simulink model "architecture1"  (R2019b)
settings: Solver=VariableStepAuto  StartTime=0.0  StopTime=10.0  RelTol=1e-3
libraries: xbsIndex_r4 x1962
settings Model: Creator=s4533087  LastModifiedBy=s4533087

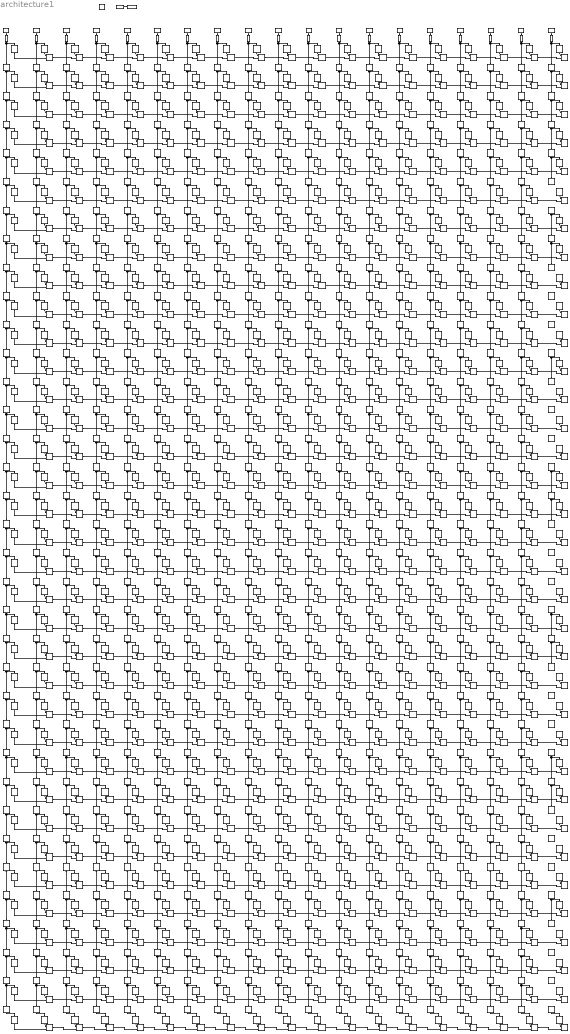
== system architecture1 ==
  " System Generator" : xbsIndex_r4/ System Generator  Tag=genX  xilinxfamily=Kintex7  part=xc7k325t  speed=-3  package=fbg676  synthesis_tool=Vivado  clock_wrapper=Clock Enables  directory=./netlist  proj_type=Vivado  Synth_file=Vivado Synthesis Defaults  Impl_file=Vivado Implementation Defaults  testbench=off  simulink_period=1  sysclk_period=10  dcm_input_clock_period=10  incr_netlist=off  trim_vbits=Everywhere in SubSystem  dbl_ovrd=According to Block Masks  core_generation=According to Block Masks  run_coregen=off  deprecated_control=off  eval_field=0  block_type=sysgen
  AddSub{1..630} (630 alike) : xbsIndex_r4/AddSub  mode=Addition  use_carryin=off  use_carryout=off  en=off  latency=0  precision=Full  arith_type=Unsigned  n_bits=16  bin_pt=14  quantization=Truncate  overflow=Wrap  use_behavioral_HDL=off  hw_selection=Fabric  pipelined=off  dbl_ovrd=off  block_type=addsub
  CMult{,1..664} (665 alike) : xbsIndex_r4/CMult  const=1  gui_display_data_type=Fixed-point  const_n_bits=16  const_bin_pt=14  float_type=Single  exp_bits=8  fraction_bits=24  en=off  latency=0  precision=User Defined  arith_type="Signed  (2's comp)"  n_bits=Wc  bin_pt=Dc  quantization=Truncate  overflow=Flag as error  use_behavioral_HDL=off  mem_type=Distributed RAM  pipeline=off  dbl_ovrd=off  block_type=cmult
  Delay{,1..645} (646 alike) : xbsIndex_r4/Delay  rst=off  infoeditControl=Selection of Reset will increase slice count due to use of real FFs and instead of SRLs  en=off  latency=1  reg_retiming=off  dbl_ovrd=off  block_type=delay
  From Workspace : FromWorkspace  VariableName=sig(:, 1)  SampleTime=0
  From Workspace1 : FromWorkspace  VariableName=sig(:, 2)  SampleTime=0
  From Workspace{2,4,6,8,10,12,14,16} (8 alike) : FromWorkspace  VariableName=sig(:, 3)  SampleTime=0
  From Workspace{3,5,7,9,11,13,15,17..18} (9 alike) : FromWorkspace  VariableName=sig(:, 4)  SampleTime=0
  Gateway In{,1..18} (19 alike) : xbsIndex_r4/Gateway In  gui_display_data_type=Fixed-point  arith_type="Signed  (2's comp)"  n_bits=W  bin_pt=D  preci_type=Single  exp_width=8  frac_width=24  rows=1  columns=1  quantization="Round  (unbiased: +/- Inf)"  overflow=Saturate  period=1  UseAsADC=off  ADCChannel='1'  interface=None  automatic_assignment=on  address_offset=hex2dec('00')  intf_name=''  intf_description=''  default_value=0  timing_constraint=None  locs_specified=off  LOCs={}  io_standard={}  inherit_from_input=off  hdl_port=on  dbl_ovrd=off  block_type=gatewayin
  Gateway Out : xbsIndex_r4/Gateway Out  inherit_from_input=off  hdl_port=on  rows=1  columns=1  UseAsDAC=off  DACChannel='1'  interface=None  automatic_assignment=on  address_offset=hex2dec('00')  intf_name=''  intf_description=''  timing_constraint=None  locs_specified=off  LOCs={}  io_standard={}  block_type=gatewayout
  To Workspace : ToWorkspace  VariableName=simout  SaveFormat=Timeseries  SampleTime=-1
  wires:
  From Workspace/1 -> Gateway In/1
  Gateway Out/1 -> To Workspace/1
  Gateway In/1 -> CMult/1, Delay/1
  Delay/1 -> CMult1/1, Delay1/1
  Delay1/1 -> CMult2/1, Delay2/1
  Delay2/1 -> CMult3/1, Delay3/1
  Delay3/1 -> CMult4/1, Delay4/1
  Delay4/1 -> CMult5/1, Delay5/1
  Delay8/1 -> CMult9/1, Delay9/1
  Delay10/1 -> CMult11/1, Delay11/1
  Delay6/1 -> CMult7/1, Delay7/1
  Delay7/1 -> CMult8/1, Delay8/1
  Delay5/1 -> CMult6/1, Delay6/1
  Delay9/1 -> CMult10/1, Delay10/1
  Delay16/1 -> CMult12/1, Delay12/1
  Delay12/1 -> CMult13/1, Delay13/1
  Delay11/1 -> CMult14/1, Delay14/1
  Delay14/1 -> CMult15/1, Delay15/1
  Delay15/1 -> CMult16/1, Delay16/1
  Delay20/1 -> CMult23/1, Delay23/1
  Delay31/1 -> CMult32/1, Delay32/1
  Delay32/1 -> CMult33/1, Delay33/1
  Delay19/1 -> CMult20/1, Delay20/1
  Delay28/1 -> CMult29/1, Delay29/1
  Delay33/1 -> CMult19/1, Delay19/1
  Delay29/1 -> CMult30/1, Delay30/1
  Delay17/1 -> CMult18/1, Delay18/1
  Delay18/1 -> CMult26/1, Delay26/1
  Delay13/1 -> CMult17/1, Delay17/1
  Delay26/1 -> CMult27/1, Delay27/1
  Delay25/1 -> CMult21/1, Delay21/1
  Delay21/1 -> CMult22/1, Delay22/1
  Delay24/1 -> CMult25/1, Delay25/1
  Delay30/1 -> CMult31/1, Delay31/1
  Delay23/1 -> CMult24/1, Delay24/1
  Delay27/1 -> CMult28/1, Delay28/1
  Delay22/1 -> CMult34/1
  Delay39/1 -> CMult44/1, Delay43/1
  CMult63/1 -> AddSub63/1
  Delay37/1 -> CMult41/1, Delay40/1
  CMult66/1 -> AddSub66/1
  CMult68/1 -> AddSub68/1
  CMult69/1 -> AddSub69/1
  Delay36/1 -> CMult38/1, Delay37/1
  Delay64/1 -> CMult67/1, Delay65/1
  CMult37/1 -> AddSub37/1
  Delay65/1 -> CMult68/1, Delay66/1
  Delay66/1 -> CMult69/1, Delay67/1
  CMult38/1 -> AddSub38/1
  Delay57/1 -> CMult64/1, Delay62/1
  CMult65/1 -> AddSub65/1
  Delay62/1 -> CMult65/1, Delay63/1
  CMult64/1 -> AddSub64/1
  CMult40/1 -> AddSub40/1
  Delay67/1 -> CMult37/1, Delay36/1
  Delay41/1 -> CMult43/1, Delay42/1
  CMult67/1 -> AddSub67/1
  Delay40/1 -> CMult42/1, Delay41/1
  CMult39/1 -> AddSub39/1
  Delay63/1 -> CMult66/1, Delay64/1
  Delay35/1 -> CMult47/1, Delay46/1
  CMult36/1 -> AddSub36/1
  Delay49/1 -> CMult63/1
  Delay34/1 -> CMult36/1, Delay35/1
  Gateway In1/1 -> CMult35/1, Delay34/1
  Delay42/1 -> CMult39/1, Delay38/1
  Delay38/1 -> CMult40/1, Delay39/1
  From Workspace1/1 -> Gateway In1/1
  CMult47/1 -> AddSub47/1
  CMult41/1 -> AddSub41/1
  CMult59/1 -> AddSub59/1
  CMult46/1 -> AddSub46/1
  Delay56/1 -> CMult59/1, Delay58/1
  CMult45/1 -> AddSub45/1
  CMult50/1 -> AddSub50/1
  Delay61/1 -> CMult46/1, Delay45/1
  Delay60/1 -> CMult62/1, Delay61/1
  CMult48/1 -> AddSub48/1
  CMult54/1 -> AddSub54/1
  CMult49/1 -> AddSub49/1
  CMult55/1 -> AddSub55/1
  Delay47/1 -> CMult51/1, Delay50/1
  CMult44/1 -> AddSub44/1
  CMult61/1 -> AddSub61/1
  Delay58/1 -> CMult60/1, Delay59/1
  Delay59/1 -> CMult61/1, Delay60/1
  Delay51/1 -> CMult53/1, Delay52/1
  CMult42/1 -> AddSub42/1
  Delay46/1 -> CMult58/1, Delay57/1
  Delay48/1 -> CMult50/1, Delay49/1
  CMult62/1 -> AddSub62/1
  Delay52/1 -> CMult49/1, Delay48/1
  CMult43/1 -> AddSub43/1
  Delay53/1 -> CMult55/1, Delay54/1
  Delay45/1 -> CMult48/1, Delay47/1
  CMult60/1 -> AddSub60/1
  CMult52/1 -> AddSub52/1
  CMult53/1 -> AddSub53/1
  Delay50/1 -> CMult52/1, Delay51/1
  CMult56/1 -> AddSub56/1
  Delay54/1 -> CMult56/1, Delay55/1
  Delay55/1 -> CMult57/1, Delay56/1
  Delay43/1 -> CMult45/1, Delay44/1
  CMult35/1 -> AddSub35/1
  CMult51/1 -> AddSub51/1
  CMult58/1 -> AddSub58/1
  CMult57/1 -> AddSub57/1
  Delay44/1 -> CMult54/1, Delay53/1
  CMult/1 -> AddSub35/2
  CMult1/1 -> AddSub36/2
  CMult2/1 -> AddSub47/2
  CMult3/1 -> AddSub58/2
  CMult4/1 -> AddSub64/2
  CMult5/1 -> AddSub65/2
  CMult6/1 -> AddSub66/2
  CMult7/1 -> AddSub67/2
  CMult8/1 -> AddSub68/2
  CMult9/1 -> AddSub69/2
  CMult10/1 -> AddSub37/2
  CMult11/1 -> AddSub38/2
  CMult14/1 -> AddSub41/2
  CMult15/1 -> AddSub42/2
  CMult16/1 -> AddSub43/2
  CMult12/1 -> AddSub39/2
  CMult13/1 -> AddSub40/2
  CMult17/1 -> AddSub44/2
  CMult18/1 -> AddSub45/2
  CMult26/1 -> AddSub54/2
  CMult27/1 -> AddSub55/2
  CMult28/1 -> AddSub56/2
  CMult29/1 -> AddSub57/2
  CMult30/1 -> AddSub59/2
  CMult31/1 -> AddSub60/2
  CMult32/1 -> AddSub61/2
  CMult33/1 -> AddSub62/2
  CMult19/1 -> AddSub46/2
  CMult20/1 -> AddSub48/2
  CMult23/1 -> AddSub51/2
  CMult24/1 -> AddSub52/2
  CMult25/1 -> AddSub53/2
  CMult21/1 -> AddSub49/2
  CMult22/1 -> AddSub50/2
  CMult34/1 -> AddSub63/2
  CMult82/1 -> AddSub13/1
  Delay90/1 -> CMult94/1, Delay92/1
  From Workspace2/1 -> Gateway In2/1
  CMult81/1 -> AddSub12/1
  CMult94/1 -> AddSub25/1
  CMult76/1 -> AddSub7/1
  Gateway In2/1 -> CMult70/1, Delay68/1
  Delay72/1 -> CMult75/1, Delay73/1
  Delay76/1 -> CMult74/1, Delay72/1
  Delay97/1 -> CMult101/1, Delay98/1
  Delay68/1 -> CMult71/1, Delay69/1
  CMult71/1 -> AddSub2/1
  Delay69/1 -> CMult82/1, Delay80/1
  Delay83/1 -> CMult98/1
  CMult102/1 -> AddSub33/1
  Delay75/1 -> CMult78/1, Delay76/1
  Delay74/1 -> CMult77/1, Delay75/1
  CMult74/1 -> AddSub5/1
  Delay101/1 -> CMult72/1, Delay70/1
  CMult75/1 -> AddSub6/1
  CMult100/1 -> AddSub31/1
  CMult99/1 -> AddSub30/1
  Delay96/1 -> CMult100/1, Delay97/1
  Delay91/1 -> CMult99/1, Delay96/1
  Delay99/1 -> CMult103/1, Delay100/1
  CMult72/1 -> AddSub3/1
  CMult73/1 -> AddSub4/1
  Delay100/1 -> CMult104/1, Delay101/1
  CMult103/1 -> AddSub34/1
  CMult101/1 -> AddSub32/1
  CMult104/1 -> AddSub70/1
  Delay98/1 -> CMult102/1, Delay99/1
  Delay71/1 -> CMult76/1, Delay74/1
  CMult98/1 -> AddSub29/1
  Delay73/1 -> CMult79/1, Delay77/1
  AddSub35/1 -> AddSub1/2
  CMult97/1 -> AddSub28/1
  Delay86/1 -> CMult84/1, Delay82/1
  Delay80/1 -> CMult93/1, Delay91/1
  Delay92/1 -> CMult95/1, Delay93/1
  CMult77/1 -> AddSub8/1
  Delay81/1 -> CMult86/1, Delay84/1
  CMult83/1 -> AddSub14/1
  CMult84/1 -> AddSub15/1
  CMult79/1 -> AddSub10/1
  CMult89/1 -> AddSub20/1
  CMult90/1 -> AddSub21/1
  Delay95/1 -> CMult81/1, Delay79/1
  CMult80/1 -> AddSub11/1
  Delay78/1 -> CMult89/1, Delay87/1
  CMult92/1 -> AddSub23/1
  CMult70/1 -> AddSub1/1
  CMult85/1 -> AddSub16/1
  CMult93/1 -> AddSub24/1
  Delay77/1 -> CMult80/1, Delay78/1
  Delay85/1 -> CMult88/1, Delay86/1
  Delay94/1 -> CMult97/1, Delay95/1
  Delay84/1 -> CMult87/1, Delay85/1
  Delay82/1 -> CMult85/1, Delay83/1
  Delay88/1 -> CMult91/1, Delay89/1
  CMult91/1 -> AddSub22/1
  Delay89/1 -> CMult92/1, Delay90/1
  Delay79/1 -> CMult83/1, Delay81/1
  Delay87/1 -> CMult90/1, Delay88/1
  Delay70/1 -> CMult73/1, Delay71/1
  CMult88/1 -> AddSub19/1
  CMult78/1 -> AddSub9/1
  CMult95/1 -> AddSub26/1
  CMult96/1 -> AddSub27/1
  CMult86/1 -> AddSub17/1
  Delay93/1 -> CMult96/1, Delay94/1
  CMult87/1 -> AddSub18/1
  AddSub36/1 -> AddSub2/2
  AddSub47/1 -> AddSub13/2
  AddSub58/1 -> AddSub24/2
  AddSub64/1 -> AddSub30/2
  AddSub65/1 -> AddSub31/2
  AddSub66/1 -> AddSub32/2
  AddSub67/1 -> AddSub33/2
  AddSub68/1 -> AddSub34/2
  AddSub69/1 -> AddSub70/2
  AddSub37/1 -> AddSub3/2
  AddSub38/1 -> AddSub4/2
  AddSub41/1 -> AddSub7/2
  AddSub42/1 -> AddSub8/2
  AddSub43/1 -> AddSub9/2
  AddSub39/1 -> AddSub5/2
  AddSub40/1 -> AddSub6/2
  AddSub44/1 -> AddSub10/2
  AddSub45/1 -> AddSub11/2
  AddSub54/1 -> AddSub20/2
  AddSub55/1 -> AddSub21/2
  AddSub56/1 -> AddSub22/2
  AddSub57/1 -> AddSub23/2
  AddSub59/1 -> AddSub25/2
  AddSub60/1 -> AddSub26/2
  AddSub61/1 -> AddSub27/2
  AddSub62/1 -> AddSub28/2
  AddSub46/1 -> AddSub12/2
  AddSub48/1 -> AddSub14/2
  AddSub51/1 -> AddSub17/2
  AddSub52/1 -> AddSub18/2
  AddSub53/1 -> AddSub19/2
  AddSub49/1 -> AddSub15/2
  AddSub50/1 -> AddSub16/2
  AddSub63/1 -> AddSub29/2
  AddSub11/1 -> AddSub73/2
  AddSub21/1 -> AddSub84/2
  AddSub3/1 -> AddSub93/2
  AddSub34/1 -> AddSub98/2
  AddSub10/1 -> AddSub72/2
  AddSub9/1 -> AddSub105/2
  AddSub17/1 -> AddSub79/2
  AddSub14/1 -> AddSub76/2
  AddSub8/1 -> AddSub104/2
  AddSub12/1 -> AddSub74/2
  AddSub15/1 -> AddSub77/2
  Delay126/1 -> CMult134/1, Delay128/1
  CMult122/1 -> AddSub75/1
  CMult134/1 -> AddSub88/1
  AddSub13/1 -> AddSub75/2
  CMult136/1 -> AddSub90/1
  Delay129/1 -> CMult136/1, Delay130/1
  CMult127/1 -> AddSub80/1
  CMult126/1 -> AddSub79/1
  Delay123/1 -> CMult130/1, Delay124/1
  CMult135/1 -> AddSub89/1
  CMult118/1 -> AddSub105/1
  Delay106/1 -> CMult113/1, Delay107/1
  CMult131/1 -> AddSub85/1
  CMult121/1 -> AddSub74/1
  Delay124/1 -> CMult131/1, Delay125/1
  Delay125/1 -> CMult132/1, Delay126/1
  Delay130/1 -> CMult137/1, Delay131/1
  CMult110/1 -> AddSub71/1
  CMult133/1 -> AddSub87/1
  Delay121/1 -> CMult128/1, Delay122/1
  Delay113/1 -> CMult120/1, Delay114/1
  CMult125/1 -> AddSub78/1
  CMult132/1 -> AddSub86/1
  CMult130/1 -> AddSub84/1
  CMult129/1 -> AddSub83/1
  Delay114/1 -> CMult129/1, Delay123/1
  CMult120/1 -> AddSub73/1
  CMult117/1 -> AddSub104/1
  Delay117/1 -> CMult126/1, Delay120/1
  CMult124/1 -> AddSub77/1
  CMult119/1 -> AddSub72/1
  CMult123/1 -> AddSub76/1
  Delay128/1 -> CMult135/1, Delay129/1
  CMult137/1 -> AddSub91/1
  Delay116/1 -> CMult133/1, Delay127/1
  Delay122/1 -> CMult124/1, Delay118/1
  Delay134/1 -> CMult107/1, Delay135/1
  Delay107/1 -> CMult116/1, Delay110/1
  Delay120/1 -> CMult127/1, Delay121/1
  CMult109/1 -> AddSub103/1
  Delay109/1 -> CMult119/1, Delay113/1
  CMult138/1 -> AddSub92/1
  CMult106/1 -> AddSub96/1
  CMult112/1 -> AddSub93/1
  Delay118/1 -> CMult125/1, Delay119/1
  Delay102/1 -> CMult109/1, Delay103/1
  CMult108/1 -> AddSub98/1
  Delay127/1 -> CMult139/1, Delay132/1
  Delay115/1 -> CMult123/1, Delay117/1
  CMult114/1 -> AddSub100/1
  Delay135/1 -> CMult108/1, Delay102/1
  CMult105/1 -> AddSub95/1
  Delay103/1 -> CMult112/1, Delay106/1
  Delay110/1 -> CMult117/1, Delay111/1
  Delay111/1 -> CMult118/1, Delay112/1
  Delay119/1 -> CMult138/1
  Delay104/1 -> CMult111/1, Delay105/1
  Delay132/1 -> CMult105/1, Delay133/1
  CMult111/1 -> AddSub82/1
  Delay112/1 -> CMult114/1, Delay108/1
  Delay108/1 -> CMult115/1, Delay109/1
  CMult113/1 -> AddSub99/1
  AddSub29/1 -> AddSub92/2
  Delay105/1 -> CMult122/1, Delay116/1
  AddSub16/1 -> AddSub78/2
  Gateway In3/1 -> CMult110/1, Delay104/1
  CMult116/1 -> AddSub102/1
  AddSub27/1 -> AddSub90/2
  AddSub30/1 -> AddSub94/2
  CMult128/1 -> AddSub81/1
  AddSub7/1 -> AddSub102/2
  Delay131/1 -> CMult121/1, Delay115/1
  AddSub4/1 -> AddSub99/2
  AddSub20/1 -> AddSub83/2
  AddSub28/1 -> AddSub91/2
  From Workspace3/1 -> Gateway In3/1
  AddSub1/1 -> AddSub71/2
  AddSub22/1 -> AddSub85/2
  AddSub19/1 -> AddSub81/2
  AddSub18/1 -> AddSub80/2
  CMult115/1 -> AddSub101/1
  CMult139/1 -> AddSub94/1
  AddSub31/1 -> AddSub95/2
  AddSub33/1 -> AddSub97/2
  AddSub32/1 -> AddSub96/2
  Delay133/1 -> CMult106/1, Delay134/1
  CMult107/1 -> AddSub97/1
  AddSub25/1 -> AddSub88/2
  AddSub70/1 -> AddSub103/2
  AddSub5/1 -> AddSub100/2
  AddSub24/1 -> AddSub87/2
  AddSub23/1 -> AddSub86/2
  AddSub2/1 -> AddSub82/2
  AddSub26/1 -> AddSub89/2
  AddSub6/1 -> AddSub101/2
  AddSub139/1 -> AddSub174/2
  AddSub135/1 -> AddSub170/2
  AddSub133/1 -> AddSub168/2
  AddSub138/1 -> AddSub173/2
  AddSub131/1 -> AddSub166/2
  AddSub136/1 -> AddSub171/2
  AddSub130/1 -> AddSub164/2
  AddSub127/1 -> AddSub161/2
  AddSub128/1 -> AddSub162/2
  AddSub122/1 -> AddSub156/2
  AddSub124/1 -> AddSub158/2
  AddSub107/1 -> AddSub146/2
  AddSub114/1 -> AddSub147/2
  AddSub142/1 -> AddSub109/2
  AddSub154/1 -> AddSub112/2
  AddSub140/1 -> AddSub175/2
  AddSub73/1 -> AddSub114/2
  AddSub93/1 -> AddSub134/2
  AddSub98/1 -> AddSub139/2
  AddSub126/1 -> AddSub160/2
  AddSub72/1 -> AddSub107/2
  AddSub105/1 -> AddSub165/2
  AddSub79/1 -> AddSub120/2
  AddSub76/1 -> AddSub117/2
  AddSub77/1 -> AddSub118/2
  CMult192/1 -> AddSub116/1
  CMult204/1 -> AddSub129/1
  AddSub75/1 -> AddSub116/2
  CMult206/1 -> AddSub131/1
  Delay197/1 -> CMult206/1, Delay198/1
  CMult197/1 -> AddSub121/1
  CMult196/1 -> AddSub120/1
  Delay191/1 -> CMult200/1, Delay192/1
  CMult205/1 -> AddSub130/1
  CMult188/1 -> AddSub165/1
  CMult201/1 -> AddSub126/1
  CMult191/1 -> AddSub115/1
  Delay192/1 -> CMult201/1, Delay193/1
  Delay193/1 -> CMult202/1, Delay194/1
  AddSub144/1 -> AddSub111/2
  Delay198/1 -> CMult207/1, Delay199/1
  Delay189/1 -> CMult198/1, Delay190/1
  Delay181/1 -> CMult190/1, Delay182/1
  CMult195/1 -> AddSub119/1
  AddSub106/1 -> AddSub145/2
  CMult202/1 -> AddSub127/1
  Delay182/1 -> CMult199/1, Delay191/1
  CMult190/1 -> AddSub114/1
  CMult194/1 -> AddSub118/1
  CMult193/1 -> AddSub117/1
  Delay196/1 -> CMult205/1, Delay197/1
  CMult207/1 -> AddSub132/1
  Delay184/1 -> CMult203/1, Delay195/1
  Delay190/1 -> CMult194/1, Delay186/1
  Delay202/1 -> CMult142/1, Delay203/1
  Delay188/1 -> CMult197/1, Delay189/1
  CMult144/1 -> AddSub144/1
  Delay177/1 -> CMult189/1, Delay181/1
  CMult141/1 -> AddSub137/1
  CMult143/1 -> AddSub139/1
  AddSub119/1 -> AddSub152/2
  CMult183/1 -> AddSub140/1
  Delay203/1 -> CMult143/1, Delay136/1
  Delay200/1 -> CMult140/1, Delay201/1
  AddSub121/1 -> AddSub155/2
  CMult184/1 -> AddSub141/1
  CMult140/1 -> AddSub136/1
  Delay137/1 -> CMult182/1, Delay174/1
  AddSub143/1 -> AddSub110/2
  Delay178/1 -> CMult187/1, Delay179/1
  Delay187/1 -> CMult208/1
  Delay172/1 -> CMult181/1, Delay173/1
  CMult181/1 -> AddSub123/1
  Delay173/1 -> CMult192/1, Delay184/1
  Delay176/1 -> CMult185/1, Delay177/1
  AddSub116/1 -> AddSub149/2
  AddSub92/1 -> AddSub133/2
  Delay201/1 -> CMult141/1, Delay202/1
  AddSub85/1 -> AddSub126/2
  AddSub101/1 -> AddSub142/2
  AddSub78/1 -> AddSub119/2
  Delay159/1 -> CMult170/1, Delay160/1
  Delay166/1 -> CMult177/1, Delay167/1
  AddSub137/1 -> AddSub172/2
  AddSub71/1 -> AddSub106/2
  Delay161/1 -> CMult172/1, Delay162/1
  AddSub104/1 -> AddSub154/2
  Delay160/1 -> CMult171/1, Delay161/1
  CMult161/1 -> AddSub148/1
  Delay194/1 -> CMult204/1, Delay196/1
  CMult171/1 -> AddSub160/1
  Delay142/1 -> CMult153/1, Delay143/1
  CMult208/1 -> AddSub133/1
  AddSub117/1 -> AddSub150/2
  CMult158/1 -> AddSub113/1
  CMult175/1 -> AddSub164/1
  Delay136/1 -> CMult144/1, Delay137/1
  CMult173/1 -> AddSub162/1
  CMult150/1 -> AddSub145/1
  CMult160/1 -> AddSub147/1
  Delay185/1 -> CMult196/1, Delay188/1
  Delay179/1 -> CMult188/1, Delay180/1
  AddSub132/1 -> AddSub167/2
  CMult169/1 -> AddSub158/1
  CMult180/1 -> AddSub106/1
  AddSub129/1 -> AddSub163/2
  CMult170/1 -> AddSub159/1
  CMult172/1 -> AddSub161/1
  CMult165/1 -> AddSub152/1
  Delay149/1 -> CMult160/1, Delay150/1
  AddSub90/1 -> AddSub131/2
  Delay157/1 -> CMult168/1, Delay158/1
  Delay175/1 -> CMult186/1, Delay178/1
  Gateway In4/1 -> CMult180/1, Delay172/1
  CMult186/1 -> AddSub143/1
  AddSub94/1 -> AddSub135/2
  CMult198/1 -> AddSub122/1
  AddSub102/1 -> AddSub143/2
  Delay199/1 -> CMult191/1, Delay183/1
  AddSub99/1 -> AddSub140/2
  AddSub83/1 -> AddSub124/2
  AddSub91/1 -> AddSub132/2
  From Workspace4/1 -> Gateway In4/1
  AddSub81/1 -> AddSub122/2
  AddSub80/1 -> AddSub121/2
  CMult147/1 -> AddSub173/1
  CMult200/1 -> AddSub125/1
  CMult155/1 -> AddSub109/1
  Delay171/1 -> CMult148/1, Delay138/1
  CMult154/1 -> AddSub108/1
  Delay151/1 -> CMult163/1, Delay153/1
  AddSub74/1 -> AddSub115/2
  CMult182/1 -> AddSub134/1
  Delay186/1 -> CMult195/1, Delay187/1
  AddSub95/1 -> AddSub136/2
  AddSub89/1 -> AddSub130/2
  Delay150/1 -> CMult169/1, Delay159/1
  AddSub86/1 -> AddSub127/2
  Delay163/1 -> CMult179/1, Delay168/1
  AddSub96/1 -> AddSub137/2
  CMult148/1 -> AddSub174/1
  CMult142/1 -> AddSub138/1
  Delay138/1 -> CMult149/1, Delay139/1
  AddSub115/1 -> AddSub148/2
  CMult178/1 -> AddSub168/1
  AddSub97/1 -> AddSub138/2
  CMult152/1 -> AddSub169/1
  CMult146/1 -> AddSub172/1
  CMult149/1 -> AddSub111/1
  Delay156/1 -> CMult167/1, Delay157/1
  AddSub123/1 -> AddSub157/2
  AddSub88/1 -> AddSub129/2
  Delay143/1 -> CMult156/1, Delay146/1
  CMult189/1 -> AddSub107/1
  AddSub103/1 -> AddSub144/2
  Delay170/1 -> CMult147/1, Delay171/1
  CMult145/1 -> AddSub171/1
  AddSub134/1 -> AddSub169/2
  AddSub165/1 -> AddSub113/2
  Delay140/1 -> CMult151/1, Delay141/1
  Delay180/1 -> CMult184/1, Delay176/1
  Delay146/1 -> CMult157/1, Delay147/1
  Gateway In5/1 -> CMult150/1, Delay140/1
  CMult179/1 -> AddSub170/1
  AddSub141/1 -> AddSub108/2
  CMult153/1 -> AddSub175/1
  AddSub84/1 -> AddSub125/2
  CMult187/1 -> AddSub154/1
  Delay144/1 -> CMult155/1, Delay145/1
  Delay141/1 -> CMult162/1, Delay152/1
  Delay168/1 -> CMult145/1, Delay169/1
  CMult168/1 -> AddSub156/1
  CMult209/1 -> AddSub135/1
  CMult156/1 -> AddSub110/1
  CMult185/1 -> AddSub142/1
  AddSub120/1 -> AddSub153/2
  Delay155/1 -> CMult178/1
  AddSub82/1 -> AddSub123/2
  CMult174/1 -> AddSub163/1
  Delay183/1 -> CMult193/1, Delay185/1
  CMult162/1 -> AddSub149/1
  Delay169/1 -> CMult146/1, Delay170/1
  Delay162/1 -> CMult174/1, Delay164/1
  CMult151/1 -> AddSub157/1
  CMult199/1 -> AddSub124/1
  CMult176/1 -> AddSub166/1
  Delay167/1 -> CMult161/1, Delay151/1
  CMult167/1 -> AddSub155/1
  Delay165/1 -> CMult176/1, Delay166/1
  CMult166/1 -> AddSub153/1
  Delay158/1 -> CMult164/1, Delay154/1
  Delay152/1 -> CMult173/1, Delay163/1
  AddSub87/1 -> AddSub128/2
  Delay148/1 -> CMult154/1, Delay144/1
  Delay195/1 -> CMult209/1, Delay200/1
  CMult177/1 -> AddSub167/1
  AddSub100/1 -> AddSub141/2
  Delay154/1 -> CMult165/1, Delay155/1
  Delay174/1 -> CMult183/1, Delay175/1
  Delay164/1 -> CMult175/1, Delay165/1
  CMult203/1 -> AddSub128/1
  AddSub118/1 -> AddSub151/2
  Delay139/1 -> CMult152/1, Delay142/1
  CMult159/1 -> AddSub146/1
  Delay145/1 -> CMult159/1, Delay149/1
  CMult164/1 -> AddSub151/1
  Delay153/1 -> CMult166/1, Delay156/1
  CMult157/1 -> AddSub112/1
  CMult163/1 -> AddSub150/1
  From Workspace5/1 -> Gateway In5/1
  AddSub125/1 -> AddSub159/2
  Delay147/1 -> CMult158/1, Delay148/1
  AddSub298/1 -> AddSub204/2
  AddSub303/1 -> AddSub209/2
  AddSub299/1 -> AddSub205/2
  AddSub291/1 -> AddSub197/2
  AddSub293/1 -> AddSub200/2
  AddSub295/1 -> AddSub201/2
  AddSub296/1 -> AddSub202/2
  AddSub287/1 -> AddSub193/2
  AddSub290/1 -> AddSub196/2
  AddSub314/1 -> AddSub220/2
  AddSub307/1 -> AddSub213/2
  AddSub310/1 -> AddSub216/2
  AddSub309/1 -> AddSub215/2
  AddSub178/1 -> AddSub223/2
  AddSub315/1 -> AddSub222/2
  AddSub181/1 -> AddSub226/2
  AddSub182/1 -> AddSub237/2
  AddSub308/1 -> AddSub214/2
  Delay287/1 -> CMult303/1, Delay289/1
  AddSub200/1 -> AddSub236/2
  CMult266/1 -> AddSub189/1
  AddSub223/1 -> AddSub186/2
  CMult278/1 -> AddSub239/1
  CMult297/1 -> AddSub237/1
  AddSub279/1 -> AddSub314/2
  AddSub273/1 -> AddSub308/2
  AddSub278/1 -> AddSub313/2
  AddSub271/1 -> AddSub306/2
  AddSub276/1 -> AddSub311/2
  AddSub267/1 -> AddSub301/2
  AddSub268/1 -> AddSub302/2
  AddSub264/1 -> AddSub298/2
  AddSub261/1 -> AddSub295/2
  Delay259/1 -> CMult288/1
  AddSub254/1 -> AddSub293/2
  AddSub265/1 -> AddSub299/2
  AddSub294/1 -> AddSub182/2
  CMult311/1 -> AddSub206/1
  CMult301/1 -> AddSub194/1
  CMult315/1 -> AddSub211/1
  CMult298/1 -> AddSub249/1
  Delay295/1 -> CMult310/1, Delay296/1
  CMult306/1 -> AddSub200/1
  CMult307/1 -> AddSub201/1
  AddSub289/1 -> AddSub195/2
  AddSub206/1 -> AddSub244/2
  AddSub222/1 -> AddSub260/2
  AddSub193/1 -> AddSub229/2
  AddSub204/1 -> AddSub241/2
  AddSub202/1 -> AddSub239/2
  AddSub211/1 -> AddSub248/2
  AddSub207/1 -> AddSub245/2
  AddSub288/1 -> AddSub194/2
  AddSub212/1 -> AddSub250/2
  AddSub214/1 -> AddSub252/2
  Delay298/1 -> CMult314/1, Delay300/1
  Delay264/1 -> CMult281/1, Delay265/1
  Delay263/1 -> CMult280/1, Delay264/1
  Delay280/1 -> CMult295/1, Delay281/1
  Delay277/1 -> CMult302/1, Delay288/1
  Delay282/1 -> CMult297/1, Delay283/1
  CMult250/1 -> AddSub217/1
  Delay291/1 -> CMult318/1
  AddSub198/1 -> AddSub235/2
  CMult293/1 -> AddSub222/1
  Delay307/1 -> CMult253/1, Delay240/1
  AddSub201/1 -> AddSub238/2
  Delay281/1 -> CMult299/1, Delay285/1
  Delay292/1 -> CMult307/1, Delay293/1
  CMult282/1 -> AddSub245/1
  CMult280/1 -> AddSub242/1
  AddSub213/1 -> AddSub251/2
  AddSub185/1 -> AddSub228/2
  Delay246/1 -> CMult263/1, Delay247/1
  AddSub169/1 -> AddSub274/2
  CMult313/1 -> AddSub208/1
  Delay270/1 -> CMult287/1, Delay271/1
  Delay268/1 -> CMult285/1, Delay269/1
  AddSub153/1 -> AddSub254/2
  AddSub150/1 -> AddSub221/2
  AddSub177/1 -> AddSub286/2
  CMult264/1 -> AddSub186/1
  Delay244/1 -> CMult261/1, Delay245/1
  CMult299/1 -> AddSub185/1
  AddSub215/1 -> AddSub253/2
  Delay274/1 -> CMult257/1, Delay275/1
  Delay247/1 -> CMult266/1, Delay250/1
  AddSub188/1 -> AddSub287/2
  AddSub292/1 -> AddSub198/2
  CMult259/1 -> AddSub190/1
  CMult262/1 -> AddSub253/1
  AddSub203/1 -> AddSub240/2
  CMult288/1 -> AddSub252/1
  AddSub194/1 -> AddSub230/2
  AddSub151/1 -> AddSub232/2
  Delay301/1 -> CMult316/1, Delay302/1
  Delay267/1 -> CMult289/1, Delay272/1
  CMult265/1 -> AddSub187/1
  From Workspace8/1 -> Gateway In8/1
  CMult257/1 -> AddSub258/1
  Delay248/1 -> CMult265/1, Delay249/1
  CMult332/1 -> AddSub210/1
  CMult344/1 -> AddSub269/1
  AddSub237/1 -> AddSub191/2
  CMult256/1 -> AddSub257/1
  AddSub184/1 -> AddSub227/2
  AddSub149/1 -> AddSub210/2
  CMult305/1 -> AddSub198/1
  Delay294/1 -> CMult304/1, Delay290/1
  AddSub275/1 -> AddSub310/2
  Delay288/1 -> CMult313/1, Delay299/1
  AddSub282/1 -> AddSub179/2
  CMult303/1 -> AddSub196/1
  AddSub224/1 -> AddSub187/2
  Delay333/1 -> CMult346/1, Delay334/1
  AddSub216/1 -> AddSub255/2
  CMult337/1 -> AddSub261/1
  CMult336/1 -> AddSub254/1
  Delay241/1 -> CMult292/1, Delay278/1
  Delay327/1 -> CMult340/1, Delay328/1
  CMult345/1 -> AddSub270/1
  CMult328/1 -> AddSub305/1
  Delay283/1 -> CMult298/1, Delay284/1
  Delay265/1 -> CMult282/1, Delay266/1
  CMult341/1 -> AddSub266/1
  Delay329/1 -> CMult342/1, Delay330/1
  CMult272/1 -> AddSub231/1
  AddSub284/1 -> AddSub181/2
  Delay297/1 -> CMult312/1, Delay298/1
  Delay334/1 -> CMult347/1, Delay335/1
  CMult268/1 -> AddSub192/1
  CMult260/1 -> AddSub227/1
  AddSub208/1 -> AddSub246/2
  Delay317/1 -> CMult330/1, Delay318/1
  CMult335/1 -> AddSub243/1
  AddSub176/1 -> AddSub285/2
  Delay296/1 -> CMult311/1, Delay297/1
  Delay318/1 -> CMult339/1, Delay327/1
  CMult330/1 -> AddSub188/1
  CMult334/1 -> AddSub232/1
  CMult333/1 -> AddSub221/1
  Delay332/1 -> CMult345/1, Delay333/1
  AddSub301/1 -> AddSub207/2
  CMult263/1 -> AddSub260/1
  CMult252/1 -> AddSub219/1
  CMult347/1 -> AddSub272/1
  Delay320/1 -> CMult343/1, Delay331/1
  Delay284/1 -> CMult294/1, Delay280/1
  AddSub285/1 -> AddSub184/2
  Delay253/1 -> CMult270/1, Delay254/1
  Delay326/1 -> CMult334/1, Delay322/1
  Delay338/1 -> CMult212/1, Delay339/1
  CMult214/1 -> AddSub284/1
  Delay313/1 -> CMult329/1, Delay317/1
  CMult211/1 -> AddSub277/1
  Delay303/1 -> CMult301/1, Delay287/1
  CMult213/1 -> AddSub279/1
  AddSub243/1 -> AddSub292/2
  CMult323/1 -> AddSub280/1
  Delay336/1 -> CMult210/1, Delay337/1
  Delay260/1 -> CMult277/1, Delay261/1
  CMult324/1 -> AddSub281/1
  AddSub297/1 -> AddSub203/2
  CMult210/1 -> AddSub276/1
  Delay205/1 -> CMult322/1, Delay310/1
  AddSub283/1 -> AddSub180/2
  Delay314/1 -> CMult327/1, Delay315/1
  Delay323/1 -> CMult348/1
  Delay308/1 -> CMult321/1, Delay309/1
  CMult321/1 -> AddSub263/1
  Delay309/1 -> CMult332/1, Delay320/1
  Delay251/1 -> CMult268/1, Delay252/1
  AddSub183/1 -> AddSub249/2
  AddSub195/1 -> AddSub231/2
  Delay312/1 -> CMult325/1, Delay313/1
  AddSub210/1 -> AddSub289/2
  AddSub313/1 -> AddSub219/2
  Delay337/1 -> CMult211/1, Delay338/1
  CMult312/1 -> AddSub207/1
  Delay278/1 -> CMult293/1, Delay279/1
  AddSub160/1 -> AddSub266/2
  AddSub220/1 -> AddSub259/2
  AddSub109/1 -> AddSub282/2
  AddSub249/1 -> AddSub192/2
  AddSub152/1 -> AddSub243/2
  Delay227/1 -> CMult240/1, Delay228/1
  Delay272/1 -> CMult255/1, Delay273/1
  AddSub311/1 -> AddSub217/2
  Delay234/1 -> CMult247/1, Delay235/1
  AddSub277/1 -> AddSub312/2
  AddSub145/1 -> AddSub176/2
  CMult251/1 -> AddSub218/1
  Delay229/1 -> CMult242/1, Delay230/1
  Delay302/1 -> CMult317/1, Delay303/1
  AddSub219/1 -> AddSub258/2
  AddSub304/1 -> AddSub211/2
  Delay228/1 -> CMult241/1, Delay229/1
  Delay290/1 -> CMult305/1, Delay291/1
  Delay330/1 -> CMult344/1, Delay332/1
  CMult241/1 -> AddSub300/1
  CMult255/1 -> AddSub256/1
  CMult348/1 -> AddSub273/1
  Delay210/1 -> CMult223/1, Delay211/1
  CMult253/1 -> AddSub220/1
  CMult228/1 -> AddSub183/1
  CMult245/1 -> AddSub304/1
  Delay204/1 -> CMult214/1, Delay205/1
  CMult243/1 -> AddSub302/1
  CMult220/1 -> AddSub285/1
  AddSub180/1 -> AddSub225/2
  CMult230/1 -> AddSub287/1
  Delay321/1 -> CMult336/1, Delay324/1
  Delay315/1 -> CMult328/1, Delay316/1
  AddSub272/1 -> AddSub307/2
  CMult302/1 -> AddSub195/1
  CMult320/1 -> AddSub176/1
  AddSub269/1 -> AddSub303/2
  Delay306/1 -> CMult252/1, Delay307/1
  CMult239/1 -> AddSub298/1
  CMult240/1 -> AddSub299/1
  CMult294/1 -> AddSub223/1
  CMult235/1 -> AddSub292/1
  CMult285/1 -> AddSub248/1
  Delay217/1 -> CMult230/1, Delay218/1
  Delay250/1 -> CMult267/1, Delay251/1
  AddSub306/1 -> AddSub212/2
  AddSub166/1 -> AddSub271/2
  Delay311/1 -> CMult326/1, Delay314/1
  Delay225/1 -> CMult238/1, Delay226/1
  Gateway In6/1 -> CMult320/1, Delay308/1
  Delay285/1 -> CMult300/1, Delay286/1
  CMult326/1 -> AddSub283/1
  AddSub226/1 -> AddSub190/2
  CMult254/1 -> AddSub226/1
  Delay249/1 -> CMult269/1, Delay253/1
  CMult274/1 -> AddSub234/1
  AddSub209/1 -> AddSub247/2
  AddSub170/1 -> AddSub275/2
  CMult338/1 -> AddSub262/1
  AddSub110/1 -> AddSub283/2
  Delay335/1 -> CMult331/1, Delay319/1
  AddSub175/1 -> AddSub280/2
  AddSub158/1 -> AddSub264/2
  AddSub167/1 -> AddSub272/2
  From Workspace6/1 -> Gateway In6/1
  AddSub179/1 -> AddSub224/2
  AddSub156/1 -> AddSub262/2
  Gateway In9/1 -> CMult260/1, Delay244/1
  CMult217/1 -> AddSub313/1
  CMult340/1 -> AddSub265/1
  CMult225/1 -> AddSub179/1
  Delay239/1 -> CMult218/1, Delay206/1
  CMult224/1 -> AddSub178/1
  Delay219/1 -> CMult233/1, Delay221/1
  AddSub148/1 -> AddSub199/2
  CMult322/1 -> AddSub274/1
  Delay322/1 -> CMult335/1, Delay323/1
  AddSub171/1 -> AddSub276/2
  AddSub164/1 -> AddSub270/2
  Delay286/1 -> CMult309/1, Delay295/1
  Delay218/1 -> CMult239/1, Delay227/1
  AddSub161/1 -> AddSub267/2
  Delay231/1 -> CMult249/1, Delay236/1
  CMult281/1 -> AddSub244/1
  AddSub172/1 -> AddSub277/2
  Delay206/1 -> CMult219/1, Delay207/1
  AddSub199/1 -> AddSub288/2
  CMult248/1 -> AddSub308/1
  AddSub173/1 -> AddSub278/2
  CMult222/1 -> AddSub309/1
  AddSub302/1 -> AddSub208/2
  CMult270/1 -> AddSub229/1
  CMult216/1 -> AddSub312/1
  CMult219/1 -> AddSub181/1
  Delay224/1 -> CMult237/1, Delay225/1
  CMult304/1 -> AddSub197/1
  AddSub263/1 -> AddSub297/2
  AddSub163/1 -> AddSub269/2
  CMult329/1 -> AddSub177/1
  Delay211/1 -> CMult226/1, Delay214/1
  CMult291/1 -> AddSub203/1
  CMult295/1 -> AddSub224/1
  AddSub111/1 -> AddSub284/2
  Delay238/1 -> CMult217/1, Delay239/1
  AddSub312/1 -> AddSub218/2
  CMult249/1 -> AddSub310/1
  AddSub281/1 -> AddSub178/2
  CMult215/1 -> AddSub311/1
  AddSub274/1 -> AddSub309/2
  Delay207/1 -> CMult222/1, Delay210/1
  AddSub305/1 -> AddSub183/2
  Delay208/1 -> CMult221/1, Delay209/1
  Delay316/1 -> CMult324/1, Delay312/1
  Delay214/1 -> CMult227/1, Delay215/1
  Gateway In7/1 -> CMult220/1, Delay208/1
  Delay305/1 -> CMult251/1, Delay306/1
  Delay209/1 -> CMult232/1, Delay220/1
  AddSub232/1 -> AddSub291/2
  CMult325/1 -> AddSub282/1
  CMult226/1 -> AddSub180/1
  CMult223/1 -> AddSub315/1
  AddSub159/1 -> AddSub265/2
  CMult327/1 -> AddSub294/1
  Delay212/1 -> CMult225/1, Delay213/1
  Delay236/1 -> CMult215/1, Delay237/1
  AddSub218/1 -> AddSub257/2
  Delay235/1 -> CMult231/1, Delay219/1
  CMult275/1 -> AddSub235/1
  CMult284/1 -> AddSub247/1
  CMult349/1 -> AddSub275/1
  CMult238/1 -> AddSub296/1
  AddSub196/1 -> AddSub233/2
  CMult289/1 -> AddSub255/1
  AddSub217/1 -> AddSub256/2
  Delay240/1 -> CMult254/1, Delay241/1
  Delay273/1 -> CMult256/1, Delay274/1
  AddSub112/1 -> AddSub294/2
  Delay275/1 -> CMult258/1, Delay242/1
  Delay266/1 -> CMult284/1, Delay268/1
  AddSub266/1 -> AddSub300/2
  AddSub174/1 -> AddSub279/2
  CMult316/1 -> AddSub212/1
  CMult314/1 -> AddSub209/1
  CMult310/1 -> AddSub205/1
  Delay324/1 -> CMult337/1, Delay325/1
  CMult277/1 -> AddSub238/1
  Delay271/1 -> CMult271/1, Delay255/1
  Delay328/1 -> CMult341/1, Delay329/1
  CMult286/1 -> AddSub250/1
  CMult309/1 -> AddSub204/1
  CMult242/1 -> AddSub301/1
  Delay276/1 -> CMult291/1, Delay277/1
  CMult271/1 -> AddSub230/1
  CMult318/1 -> AddSub214/1
  Delay223/1 -> CMult248/1
  Delay215/1 -> CMult228/1, Delay216/1
  CMult244/1 -> AddSub303/1
  Delay319/1 -> CMult333/1, Delay321/1
  AddSub225/1 -> AddSub189/2
  CMult232/1 -> AddSub289/1
  Delay237/1 -> CMult216/1, Delay238/1
  Delay262/1 -> CMult274/1, Delay258/1
  CMult221/1 -> AddSub297/1
  CMult339/1 -> AddSub264/1
  CMult212/1 -> AddSub278/1
  CMult218/1 -> AddSub314/1
  CMult283/1 -> AddSub246/1
  Delay230/1 -> CMult244/1, Delay232/1
  CMult276/1 -> AddSub236/1
  AddSub168/1 -> AddSub273/2
  Delay255/1 -> CMult273/1, Delay257/1
  CMult237/1 -> AddSub295/1
  CMult300/1 -> AddSub193/1
  CMult269/1 -> AddSub228/1
  Delay269/1 -> CMult286/1, Delay270/1
  AddSub197/1 -> AddSub234/2
  CMult317/1 -> AddSub213/1
  AddSub221/1 -> AddSub290/2
  Delay220/1 -> CMult243/1, Delay231/1
  AddSub162/1 -> AddSub268/2
  AddSub108/1 -> AddSub281/2
  AddSub300/1 -> AddSub206/2
  CMult258/1 -> AddSub259/1
  CMult247/1 -> AddSub307/1
  CMult229/1 -> AddSub286/1
  Delay213/1 -> CMult229/1, Delay217/1
  CMult234/1 -> AddSub291/1
  Delay221/1 -> CMult236/1, Delay224/1
  CMult227/1 -> AddSub182/1
  Delay304/1 -> CMult250/1, Delay305/1
  AddSub146/1 -> AddSub177/2
  Delay331/1 -> CMult349/1, Delay336/1
  Delay216/1 -> CMult224/1, Delay212/1
  Delay258/1 -> CMult275/1, Delay259/1
  CMult331/1 -> AddSub199/1
  CMult233/1 -> AddSub290/1
  CMult279/1 -> AddSub241/1
  CMult273/1 -> AddSub233/1
  CMult267/1 -> AddSub191/1
  CMult290/1 -> AddSub184/1
  AddSub270/1 -> AddSub304/2
  Delay222/1 -> CMult235/1, Delay223/1
  Delay293/1 -> CMult308/1, Delay294/1
  Delay310/1 -> CMult323/1, Delay311/1
  CMult292/1 -> AddSub215/1
  Delay257/1 -> CMult276/1, Delay260/1
  Delay226/1 -> CMult234/1, Delay222/1
  AddSub157/1 -> AddSub263/2
  Delay300/1 -> CMult315/1, Delay301/1
  Delay252/1 -> CMult264/1, Delay248/1
  CMult246/1 -> AddSub306/1
  AddSub147/1 -> AddSub188/2
  Delay242/1 -> CMult259/1, Delay243/1
  Delay339/1 -> CMult213/1, Delay204/1
  CMult287/1 -> AddSub251/1
  Delay254/1 -> CMult279/1, Delay263/1
  Delay299/1 -> CMult319/1, Delay304/1
  CMult231/1 -> AddSub288/1
  CMult296/1 -> AddSub225/1
  AddSub280/1 -> AddSub315/2
  CMult236/1 -> AddSub293/1
  CMult319/1 -> AddSub216/1
  Gateway In8/1 -> CMult290/1, Delay276/1
  Delay279/1 -> CMult296/1, Delay282/1
  AddSub262/1 -> AddSub296/2
  Delay232/1 -> CMult245/1, Delay233/1
  CMult343/1 -> AddSub268/1
  Delay261/1 -> CMult278/1, Delay262/1
  Delay233/1 -> CMult246/1, Delay234/1
  CMult342/1 -> AddSub267/1
  CMult261/1 -> AddSub240/1
  AddSub286/1 -> AddSub185/2
  Delay245/1 -> CMult272/1, Delay256/1
  Delay243/1 -> CMult262/1, Delay246/1
  Delay289/1 -> CMult306/1, Delay292/1
  AddSub113/1 -> AddSub305/2
  AddSub155/1 -> AddSub261/2
  Delay256/1 -> CMult283/1, Delay267/1
  Delay325/1 -> CMult338/1, Delay326/1
  CMult308/1 -> AddSub202/1
  From Workspace7/1 -> Gateway In7/1
  CMult346/1 -> AddSub271/1
  From Workspace9/1 -> Gateway In9/1
  AddSub205/1 -> AddSub242/2
  AddSub329/1 -> AddSub520/2
  AddSub331/1 -> AddSub532/2
  AddSub378/1 -> AddSub496/2
  AddSub330/1 -> AddSub521/2
  AddSub371/1 -> AddSub440/2
  AddSub375/1 -> AddSub476/2
  AddSub370/1 -> AddSub426/2
  AddSub384/1 -> AddSub501/2
  AddSub395/1 -> AddSub511/2
  AddSub393/1 -> AddSub510/2
  AddSub397/1 -> AddSub513/2
  AddSub388/1 -> AddSub506/2
  AddSub386/1 -> AddSub503/2
  AddSub391/1 -> AddSub508/2
  AddSub379/1 -> AddSub497/2
  AddSub396/1 -> AddSub512/2
  AddSub392/1 -> AddSub509/2
  AddSub368/1 -> AddSub402/2
  AddSub332/1 -> AddSub545/2
  AddSub434/1 -> AddSub475/2
  From Workspace17/1 -> Gateway In17/1
  From Workspace15/1 -> Gateway In15/1
  Delay496/1 -> CMult533/1, Delay507/1
  CMult558/1 -> AddSub431/1
  AddSub387/1 -> AddSub504/2
  Delay483/1 -> CMult512/1, Delay486/1
  AddSub523/1 -> AddSub411/2
  Delay529/1 -> CMult556/1, Delay532/1
  Delay472/1 -> CMult495/1, Delay473/1
  Delay473/1 -> CMult496/1, Delay474/1
  CMult593/1 -> AddSub503/1
  CMult486/1 -> AddSub531/1
  Delay519/1 -> CMult546/1, Delay522/1
  Gateway In16/1 -> CMult540/1, Delay516/1
  CMult546/1 -> AddSub456/1
  Delay539/1 -> CMult569/1, Delay544/1
  Delay494/1 -> CMult529/1, Delay503/1
  CMult537/1 -> AddSub485/1
  Delay482/1 -> CMult509/1, Delay483/1
  Delay579/1 -> CMult463/1, Delay444/1
  Delay462/1 -> CMult485/1, Delay463/1
  CMult529/1 -> AddSub474/1
  CMult517/1 -> AddSub418/1
  CMult581/1 -> AddSub426/1
  AddSub506/1 -> AddSub544/2
  Delay498/1 -> CMult525/1, Delay499/1
  Delay453/1 -> CMult479/1, Delay457/1
  CMult477/1 -> AddSub408/1
  CMult508/1 -> AddSub493/1
  AddSub540/1 -> AddSub435/2
  Delay460/1 -> CMult493/1, Delay471/1
  CMult487/1 -> AddSub533/1
  CMult550/1 -> AddSub420/1
  AddSub452/1 -> AddSub528/2
  CMult567/1 -> AddSub443/1
  CMult519/1 -> AddSub459/1
  CMult481/1 -> AddSub525/1
  Delay495/1 -> CMult523/1, Delay497/1
  CMult589/1 -> AddSub499/1
  AddSub517/1 -> AddSub556/2
  CMult471/1 -> AddSub535/1
  Delay477/1 -> CMult466/1, Delay478/1
  AddSub456/1 -> AddSub415/2
  Delay463/1 -> CMult498/1
  CMult494/1 -> AddSub543/1
  Delay455/1 -> CMult478/1, Delay456/1
  CMult536/1 -> AddSub484/1
  CMult559/1 -> AddSub433/1
  Delay516/1 -> CMult541/1, Delay517/1
  Delay511/1 -> CMult521/1, Delay495/1
  Delay506/1 -> CMult534/1, Delay508/1
  AddSub501/1 -> AddSub540/2
  CMult566/1 -> AddSub442/1
  Delay480/1 -> CMult504/1, Delay481/1
  AddSub447/1 -> AddSub490/2
  AddSub423/1 -> AddSub465/2
  CMult488/1 -> AddSub534/1
  AddSub390/1 -> AddSub507/2
  CMult525/1 -> AddSub467/1
  CMult575/1 -> AddSub519/1
  Delay545/1 -> CMult501/1, Delay546/1
  Delay492/1 -> CMult514/1, Delay488/1
  Delay448/1 -> CMult471/1, Delay449/1
  Delay556/1 -> CMult574/1, Delay552/1
  CMult465/1 -> AddSub552/1
  CMult499/1 -> AddSub551/1
  AddSub553/1 -> AddSub448/2
  CMult596/1 -> AddSub507/1
  CMult545/1 -> AddSub455/1
  CMult579/1 -> AddSub402/1
  Delay464/1 -> CMult487/1, Delay465/1
  CMult466/1 -> AddSub553/1
  CMult469/1 -> AddSub407/1
  Delay466/1 -> CMult484/1, Delay462/1
  CMult472/1 -> AddSub549/1
  CMult520/1 -> AddSub460/1
  AddSub542/1 -> AddSub437/2
  CMult531/1 -> AddSub477/1
  AddSub426/1 -> AddSub525/2
  CMult523/1 -> AddSub465/1
  CMult498/1 -> AddSub548/1
  Delay471/1 -> CMult499/1, Delay476/1
  Delay446/1 -> CMult469/1, Delay447/1
  Delay458/1 -> CMult489/1, Delay467/1
  CMult590/1 -> AddSub500/1
  CMult474/1 -> AddSub403/1
  Delay533/1 -> CMult558/1, Delay534/1
  Delay479/1 -> CMult468/1, Delay446/1
  From Workspace14/1 -> Gateway In14/1
  Delay564/1 -> CMult587/1, Delay565/1
  Delay489/1 -> CMult519/1, Delay493/1
  Delay497/1 -> CMult526/1, Delay500/1
  CMult588/1 -> AddSub497/1
  CMult504/1 -> AddSub457/1
  Gateway In14/1 -> CMult570/1, Delay548/1
  CMult576/1 -> AddSub520/1
  Delay525/1 -> CMult550/1, Delay526/1
  Delay465/1 -> CMult488/1, Delay466/1
  AddSub546/1 -> AddSub442/2
  Delay457/1 -> CMult480/1, Delay458/1
  CMult535/1 -> AddSub481/1
  Delay461/1 -> CMult486/1, Delay464/1
  CMult489/1 -> AddSub536/1
  CMult570/1 -> AddSub401/1
  CMult552/1 -> AddSub422/1
  Delay555/1 -> CMult578/1, Delay556/1
  CMult480/1 -> AddSub524/1
  CMult493/1 -> AddSub542/1
  CMult560/1 -> AddSub434/1
  AddSub380/1 -> AddSub498/2
  Delay444/1 -> CMult464/1, Delay445/1
  Delay485/1 -> CMult522/1, Delay496/1
  AddSub406/1 -> AddSub456/2
  AddSub326/1 -> AddSub518/2
  CMult505/1 -> AddSub490/1
  CMult491/1 -> AddSub540/1
  AddSub449/1 -> AddSub492/2
  Delay530/1 -> CMult555/1, Delay531/1
  AddSub398/1 -> AddSub514/2
  Delay570/1 -> CMult594/1, Delay572/1
  Delay474/1 -> CMult497/1, Delay475/1
  Delay518/1 -> CMult543/1, Delay519/1
  AddSub482/1 -> AddSub419/2
  Delay577/1 -> CMult461/1, Delay578/1
  Delay552/1 -> CMult575/1, Delay553/1
  AddSub409/1 -> AddSub482/2
  AddSub554/1 -> AddSub449/2
  CMult571/1 -> AddSub498/1
  Delay563/1 -> CMult598/1
  AddSub520/1 -> AddSub406/2
  CMult574/1 -> AddSub518/1
  CMult460/1 -> AddSub512/1
  CMult490/1 -> AddSub537/1
  AddSub544/1 -> AddSub441/2
  CMult463/1 -> AddSub515/1
  Delay550/1 -> CMult573/1, Delay551/1
  AddSub497/1 -> AddSub534/2
  AddSub476/1 -> AddSub530/2
  Delay578/1 -> CMult462/1, Delay579/1
  Delay493/1 -> CMult520/1, Delay494/1
  AddSub440/1 -> AddSub526/2
  Delay524/1 -> CMult544/1, Delay520/1
  Delay559/1 -> CMult583/1, Delay561/1
  CMult597/1 -> AddSub508/1
  Delay467/1 -> CMult490/1, Delay468/1
  Delay572/1 -> CMult595/1, Delay573/1
  CMult568/1 -> AddSub444/1
  AddSub541/1 -> AddSub436/2
  CMult513/1 -> AddSub495/1
  Delay560/1 -> CMult593/1, Delay571/1
  CMult584/1 -> AddSub464/1
  Delay554/1 -> CMult577/1, Delay555/1
  CMult496/1 -> AddSub546/1
  CMult580/1 -> AddSub414/1
  AddSub404/1 -> AddSub455/2
  Delay536/1 -> CMult561/1, Delay537/1
  CMult467/1 -> AddSub554/1
  Delay515/1 -> CMult508/1, Delay482/1
  CMult583/1 -> AddSub452/1
  CMult510/1 -> AddSub458/1
  Delay557/1 -> CMult580/1, Delay558/1
  AddSub437/1 -> AddSub479/2
  CMult518/1 -> AddSub419/1
  CMult585/1 -> AddSub476/1
  AddSub521/1 -> AddSub407/2
  CMult591/1 -> AddSub501/1
  Delay569/1 -> CMult592/1, Delay570/1
  Delay523/1 -> CMult548/1, Delay524/1
  Delay481/1 -> CMult542/1, Delay518/1
  Delay567/1 -> CMult590/1, Delay568/1
  Delay573/1 -> CMult596/1, Delay574/1
  CMult587/1 -> AddSub496/1
  AddSub519/1 -> AddSub404/2
  Delay512/1 -> CMult505/1, Delay513/1
  AddSub511/1 -> AddSub551/2
  CMult484/1 -> AddSub529/1
  CMult506/1 -> AddSub491/1
  AddSub410/1 -> AddSub458/2
  AddSub469/1 -> AddSub418/2
  From Workspace16/1 -> Gateway In16/1
  CMult515/1 -> AddSub413/1
  AddSub530/1 -> AddSub425/2
  AddSub432/1 -> AddSub473/2
  CMult514/1 -> AddSub412/1
  Delay514/1 -> CMult507/1, Delay515/1
  AddSub402/1 -> AddSub523/2
  CMult530/1 -> AddSub475/1
  Delay532/1 -> CMult557/1, Delay533/1
  CMult572/1 -> AddSub510/1
  Delay459/1 -> CMult483/1, Delay461/1
  AddSub401/1 -> AddSub522/2
  AddSub578/1 -> AddSub344/2
  AddSub583/1 -> AddSub349/2
  AddSub579/1 -> AddSub345/2
  CMult569/1 -> AddSub446/1
  AddSub571/1 -> AddSub337/2
  CMult555/1 -> AddSub425/1
  AddSub573/1 -> AddSub340/2
  AddSub575/1 -> AddSub341/2
  AddSub576/1 -> AddSub342/2
  AddSub422/1 -> AddSub463/2
  AddSub567/1 -> AddSub333/2
  AddSub594/1 -> AddSub360/2
  AddSub411/1 -> AddSub459/2
  AddSub587/1 -> AddSub353/2
  AddSub589/1 -> AddSub355/2
  AddSub318/1 -> AddSub363/2
  Delay491/1 -> CMult518/1, Delay492/1
  AddSub595/1 -> AddSub362/2
  Delay484/1 -> CMult511/1, Delay485/1
  Delay553/1 -> CMult579/1, Delay557/1
  AddSub321/1 -> AddSub366/2
  AddSub322/1 -> AddSub377/2
  AddSub588/1 -> AddSub354/2
  AddSub381/1 -> AddSub499/2
  AddSub508/1 -> AddSub547/2
  Delay575/1 -> CMult581/1, Delay559/1
  CMult495/1 -> AddSub544/1
  AddSub522/1 -> AddSub410/2
  AddSub340/1 -> AddSub376/2
  AddSub363/1 -> AddSub326/2
  CMult418/1 -> AddSub379/1
  CMult543/1 -> AddSub453/1
  CMult437/1 -> AddSub377/1
  AddSub559/1 -> AddSub594/2
  AddSub558/1 -> AddSub593/2
  AddSub505/1 -> AddSub586/2
  AddSub550/1 -> AddSub591/2
  Delay507/1 -> CMult539/1, Delay512/1
  AddSub461/1 -> AddSub581/2
  Delay500/1 -> CMult527/1, Delay501/1
  AddSub472/1 -> AddSub582/2
  Delay395/1 -> CMult428/1
  AddSub405/1 -> AddSub575/2
  AddSub439/1 -> AddSub579/2
  CMult441/1 -> AddSub334/1
  CMult455/1 -> AddSub351/1
  CMult509/1 -> AddSub417/1
  CMult438/1 -> AddSub389/1
  Delay431/1 -> CMult450/1, Delay432/1
  CMult446/1 -> AddSub340/1
  AddSub569/1 -> AddSub335/2
  CMult522/1 -> AddSub463/1
  AddSub346/1 -> AddSub384/2
  AddSub362/1 -> AddSub400/2
  AddSub333/1 -> AddSub369/2
  CMult485/1 -> AddSub530/1
  AddSub344/1 -> AddSub381/2
  AddSub342/1 -> AddSub379/2
  AddSub351/1 -> AddSub388/2
  AddSub568/1 -> AddSub334/2
  AddSub347/1 -> AddSub385/2
  Delay468/1 -> CMult491/1, Delay469/1
  AddSub352/1 -> AddSub390/2
  AddSub354/1 -> AddSub392/2
  Delay434/1 -> CMult454/1, Delay436/1
  Delay400/1 -> CMult421/1, Delay401/1
  CMult577/1 -> AddSub532/1
  CMult527/1 -> AddSub470/1
  Delay399/1 -> CMult420/1, Delay400/1
  CMult479/1 -> AddSub523/1
  CMult511/1 -> AddSub473/1
  Delay416/1 -> CMult435/1, Delay417/1
  Delay418/1 -> CMult437/1, Delay419/1
  Delay548/1 -> CMult571/1, Delay549/1
  CMult390/1 -> AddSub357/1
  Delay427/1 -> CMult458/1
  CMult483/1 -> AddSub528/1
  AddSub338/1 -> AddSub375/2
  Delay488/1 -> CMult515/1, Delay489/1
  CMult433/1 -> AddSub362/1
  CMult478/1 -> AddSub409/1
  Delay445/1 -> CMult572/1, Delay550/1
  Delay443/1 -> CMult393/1, Delay376/1
  AddSub341/1 -> AddSub378/2
  CMult599/1 -> AddSub511/1
  Delay417/1 -> CMult439/1, Delay421/1
  Delay428/1 -> CMult447/1, Delay429/1
  Delay389/1 -> CMult410/1, Delay390/1
  CMult415/1 -> AddSub375/1
  CMult424/1 -> AddSub387/1
  CMult422/1 -> AddSub385/1
  CMult540/1 -> AddSub410/1
  CMult420/1 -> AddSub382/1
  CMult554/1 -> AddSub424/1
  AddSub353/1 -> AddSub391/2
  AddSub325/1 -> AddSub368/2
  AddSub494/1 -> AddSub584/2
  CMult430/1 -> AddSub324/1
  Delay376/1 -> CMult394/1, Delay377/1
  CMult408/1 -> AddSub332/1
  CMult425/1 -> AddSub388/1
  CMult429/1 -> AddSub395/1
  AddSub336/1 -> AddSub373/2
  AddSub498/1 -> AddSub535/2
  Delay382/1 -> CMult403/1, Delay383/1
  CMult421/1 -> AddSub384/1
  CMult578/1 -> AddSub545/1
  Delay387/1 -> CMult408/1, Delay388/1
  AddSub242/1 -> AddSub439/2
  AddSub253/1 -> AddSub538/2
  Delay406/1 -> CMult427/1, Delay407/1
  CMult453/1 -> AddSub348/1
  Delay404/1 -> CMult425/1, Delay405/1
  AddSub259/1 -> AddSub559/2
  CMult456/1 -> AddSub352/1
  Delay414/1 -> CMult433/1, Delay415/1
  CMult524/1 -> AddSub466/1
  AddSub228/1 -> AddSub317/2
  Delay425/1 -> CMult446/1, Delay428/1
  AddSub535/1 -> AddSub432/2
  AddSub192/1 -> AddSub585/2
  AddSub454/1 -> AddSub412/2
  CMult451/1 -> AddSub346/1
  CMult516/1 -> AddSub415/1
  Delay527/1 -> CMult553/1, Delay529/1
  AddSub414/1 -> AddSub524/2
  AddSub548/1 -> AddSub444/2
  AddSub547/1 -> AddSub443/2
  AddSub524/1 -> AddSub420/2
  AddSub407/1 -> AddSub457/2
  Delay510/1 -> CMult537/1, Delay511/1
  AddSub556/1 -> AddSub453/2
  AddSub590/1 -> AddSub356/2
  AddSub549/1 -> AddSub445/2
  AddSub551/1 -> AddSub446/2
  CMult470/1 -> AddSub522/1
  AddSub428/1 -> AddSub578/2
  AddSub533/1 -> AddSub430/2
  AddSub527/1 -> AddSub588/2
  Delay544/1 -> CMult500/1, Delay545/1
  AddSub536/1 -> AddSub433/2
  AddSub441/1 -> AddSub481/2
  CMult507/1 -> AddSub492/1
  AddSub442/1 -> AddSub484/2
  AddSub431/1 -> AddSub471/2
  AddSub444/1 -> AddSub486/2
  AddSub525/1 -> AddSub421/2
  CMult468/1 -> AddSub555/1
  AddSub436/1 -> AddSub478/2
  Delay423/1 -> CMult443/1, Delay425/1
  AddSub433/1 -> AddSub474/2
  AddSub453/1 -> AddSub495/2
  AddSub435/1 -> AddSub477/2
  Delay413/1 -> CMult442/1, Delay424/1
  CMult556/1 -> AddSub429/1
  CMult548/1 -> AddSub482/1
  Delay508/1 -> CMult535/1, Delay509/1
  CMult565/1 -> AddSub441/1
  CMult406/1 -> AddSub329/1
  AddSub496/1 -> AddSub533/2
  AddSub488/1 -> AddSub531/2
  Delay499/1 -> CMult538/1
  AddSub503/1 -> AddSub542/2
  Delay450/1 -> CMult473/1, Delay451/1
  Delay487/1 -> CMult516/1, Delay490/1
  AddSub532/1 -> AddSub408/2
  AddSub574/1 -> AddSub322/2
  AddSub514/1 -> AddSub554/2
  CMult482/1 -> AddSub526/1
  CMult528/1 -> AddSub471/1
  CMult534/1 -> AddSub480/1
  CMult447/1 -> AddSub341/1
  AddSub236/1 -> AddSub394/2
  AddSub233/1 -> AddSub361/2
  Delay476/1 -> CMult465/1, Delay477/1
  AddSub455/1 -> AddSub413/2
  Delay542/1 -> CMult567/1, Delay543/1
  AddSub317/1 -> AddSub566/2
  CMult404/1 -> AddSub326/1
  Delay380/1 -> CMult401/1, Delay381/1
  Delay534/1 -> CMult554/1, Delay530/1
  AddSub545/1 -> AddSub409/2
  CMult439/1 -> AddSub325/1
  AddSub355/1 -> AddSub393/2
  Delay410/1 -> CMult397/1, Delay411/1
  AddSub572/1 -> AddSub338/2
  AddSub328/1 -> AddSub567/2
  Delay383/1 -> CMult406/1, Delay386/1
  CMult492/1 -> AddSub541/1
  CMult532/1 -> AddSub478/1
  AddSub448/1 -> AddSub491/2
  CMult399/1 -> AddSub330/1
  CMult521/1 -> AddSub462/1
  CMult402/1 -> AddSub393/1
  CMult428/1 -> AddSub392/1
  AddSub343/1 -> AddSub380/2
  AddSub334/1 -> AddSub370/2
  AddSub234/1 -> AddSub372/2
  Delay437/1 -> CMult456/1, Delay438/1
  Delay403/1 -> CMult429/1, Delay408/1
  Delay478/1 -> CMult467/1, Delay479/1
  AddSub515/1 -> AddSub555/2
  Delay540/1 -> CMult565/1, Delay541/1
  CMult405/1 -> AddSub327/1
  From Workspace12/1 -> Gateway In12/1
  Delay384/1 -> CMult405/1, Delay385/1
  CMult397/1 -> AddSub398/1
  CMult612/1 -> AddSub350/1
  CMult624/1 -> AddSub483/1
  AddSub377/1 -> AddSub331/2
  AddSub385/1 -> AddSub502/2
  CMult396/1 -> AddSub397/1
  CMult462/1 -> AddSub514/1
  CMult501/1 -> AddSub448/1
  AddSub324/1 -> AddSub367/2
  AddSub231/1 -> AddSub350/2
  CMult445/1 -> AddSub338/1
  Delay430/1 -> CMult444/1, Delay426/1
  AddSub539/1 -> AddSub590/2
  Delay424/1 -> CMult453/1, Delay435/1
  AddSub562/1 -> AddSub319/2
  CMult443/1 -> AddSub336/1
  Delay469/1 -> CMult492/1, Delay470/1
  AddSub364/1 -> AddSub327/2
  AddSub327/1 -> AddSub519/2
  AddSub356/1 -> AddSub395/2
  Delay605/1 -> CMult626/1, Delay606/1
  CMult617/1 -> AddSub405/1
  Delay377/1 -> CMult432/1, Delay414/1
  CMult616/1 -> AddSub394/1
  Delay599/1 -> CMult620/1, Delay600/1
  CMult625/1 -> AddSub494/1
  CMult608/1 -> AddSub585/1
  AddSub446/1 -> AddSub489/2
  CMult598/1 -> AddSub509/1
  Delay541/1 -> CMult566/1, Delay542/1
  Delay419/1 -> CMult438/1, Delay420/1
  Delay401/1 -> CMult422/1, Delay402/1
  CMult621/1 -> AddSub450/1
  Delay601/1 -> CMult622/1, Delay602/1
  Delay505/1 -> CMult532/1, Delay506/1
  CMult412/1 -> AddSub371/1
  AddSub564/1 -> AddSub321/2
  Delay433/1 -> CMult452/1, Delay434/1
  Delay606/1 -> CMult627/1, Delay607/1
  AddSub429/1 -> AddSub468/2
  CMult400/1 -> AddSub367/1
  AddSub348/1 -> AddSub386/2
  AddSub510/1 -> AddSub549/2
  AddSub408/1 -> AddSub469/2
  Delay543/1 -> CMult551/1, Delay527/1
  Delay589/1 -> CMult610/1, Delay590/1
  AddSub500/1 -> AddSub537/2
  AddSub518/1 -> AddSub403/2
  AddSub316/1 -> AddSub565/2
  CMult615/1 -> AddSub383/1
  Delay432/1 -> CMult451/1, Delay433/1
  CMult610/1 -> AddSub328/1
  CMult614/1 -> AddSub372/1
  CMult613/1 -> AddSub361/1
  Delay604/1 -> CMult625/1, Delay605/1
  AddSub581/1 -> AddSub347/2
  Delay452/1 -> CMult475/1, Delay453/1
  CMult403/1 -> AddSub400/1
  CMult392/1 -> AddSub359/1
  CMult627/1 -> AddSub516/1
  CMult544/1 -> AddSub454/1
  Delay592/1 -> CMult623/1, Delay603/1
  Delay449/1 -> CMult482/1, Delay460/1
  Delay420/1 -> CMult434/1, Delay416/1
  AddSub565/1 -> AddSub324/2
  Delay546/1 -> CMult502/1, Delay547/1
  Delay598/1 -> CMult614/1, Delay594/1
  Delay610/1 -> CMult352/1, Delay611/1
  CMult354/1 -> AddSub564/1
  CMult541/1 -> AddSub432/1
  CMult533/1 -> AddSub479/1
  Delay585/1 -> CMult609/1, Delay589/1
  CMult497/1 -> AddSub547/1
  Delay566/1 -> CMult584/1, Delay562/1
  CMult351/1 -> AddSub557/1
  Delay439/1 -> CMult441/1, Delay423/1
  CMult353/1 -> AddSub559/1
  AddSub383/1 -> AddSub572/2
  CMult603/1 -> AddSub560/1
  CMult551/1 -> AddSub421/1
  Delay396/1 -> CMult417/1, Delay397/1
  CMult473/1 -> AddSub556/1
  CMult604/1 -> AddSub561/1
  AddSub577/1 -> AddSub343/2
  AddSub543/1 -> AddSub438/2
  CMult350/1 -> AddSub550/1
  AddSub563/1 -> AddSub320/2
  Delay341/1 -> CMult602/1, Delay582/1
  Delay451/1 -> CMult476/1, Delay454/1
  Delay586/1 -> CMult607/1, Delay587/1
  Delay571/1 -> CMult599/1, Delay576/1
  CMult542/1 -> AddSub445/1
  AddSub529/1 -> AddSub424/2
  Delay595/1 -> CMult628/1
  CMult601/1 -> AddSub427/1
  Delay581/1 -> CMult612/1, Delay592/1
  AddSub323/1 -> AddSub389/2
  AddSub528/1 -> AddSub423/2
  CMult561/1 -> AddSub435/1
  AddSub335/1 -> AddSub371/2
  Delay584/1 -> CMult605/1, Delay585/1
  AddSub350/1 -> AddSub569/2
  AddSub593/1 -> AddSub359/2
  AddSub509/1 -> AddSub548/2
  Delay609/1 -> CMult351/1, Delay610/1
  CMult452/1 -> AddSub347/1
  AddSub570/1 -> AddSub336/2
  CMult475/1 -> AddSub404/1
  AddSub360/1 -> AddSub399/2
  AddSub244/1 -> AddSub450/2
  Delay520/1 -> CMult545/1, Delay521/1
  Delay558/1 -> CMult589/1, Delay567/1
  Delay590/1 -> CMult619/1, Delay599/1
  AddSub187/1 -> AddSub562/2
  AddSub235/1 -> AddSub383/2
  AddSub537/1 -> AddSub434/2
  AddSub389/1 -> AddSub332/2
  AddSub513/1 -> AddSub553/2
  AddSub591/1 -> AddSub357/2
  Delay503/1 -> CMult530/1, Delay504/1
  CMult553/1 -> AddSub423/1
  Delay370/1 -> CMult387/1, Delay371/1
  AddSub557/1 -> AddSub592/2
  CMult391/1 -> AddSub358/1
  Delay574/1 -> CMult597/1, Delay575/1
  AddSub227/1 -> AddSub316/2
  Delay438/1 -> CMult457/1, Delay439/1
  AddSub584/1 -> AddSub351/2
  AddSub359/1 -> AddSub398/2
  Delay365/1 -> CMult382/1, Delay366/1
  AddSub512/1 -> AddSub552/2
  Delay504/1 -> CMult531/1, Delay505/1
  CMult594/1 -> AddSub504/1
  Delay364/1 -> CMult381/1, Delay365/1
  Delay475/1 -> CMult481/1, Delay459/1
  Delay426/1 -> CMult445/1, Delay427/1
  Delay602/1 -> CMult624/1, Delay604/1
  CMult539/1 -> AddSub489/1
  AddSub399/1 -> AddSub515/2
  CMult381/1 -> AddSub580/1
  Delay538/1 -> CMult564/1, Delay540/1
  CMult393/1 -> AddSub360/1
  Delay346/1 -> CMult363/1, Delay347/1
  CMult628/1 -> AddSub527/1
  CMult395/1 -> AddSub396/1
  Delay565/1 -> CMult588/1, Delay566/1
  Delay363/1 -> CMult380/1, Delay364/1
  Delay408/1 -> CMult395/1, Delay409/1
  Delay509/1 -> CMult536/1, Delay510/1
  CMult368/1 -> AddSub323/1
  CMult385/1 -> AddSub584/1
  Delay340/1 -> CMult354/1, Delay341/1
  AddSub499/1 -> AddSub536/2
  CMult383/1 -> AddSub582/1
  AddSub373/1 -> AddSub452/2
  CMult360/1 -> AddSub565/1
  AddSub320/1 -> AddSub365/2
  CMult370/1 -> AddSub567/1
  CMult526/1 -> AddSub468/1
  Delay593/1 -> CMult616/1, Delay596/1
  AddSub516/1 -> AddSub587/2
  Delay587/1 -> CMult608/1, Delay588/1
  CMult442/1 -> AddSub335/1
  CMult600/1 -> AddSub316/1
  AddSub483/1 -> AddSub583/2
  CMult502/1 -> AddSub449/1
  CMult379/1 -> AddSub578/1
  Delay442/1 -> CMult392/1, Delay443/1
  CMult434/1 -> AddSub363/1
  CMult380/1 -> AddSub579/1
  CMult375/1 -> AddSub572/1
  Delay353/1 -> CMult370/1, Delay354/1
  Delay386/1 -> CMult407/1, Delay387/1
  AddSub586/1 -> AddSub352/2
  AddSub250/1 -> AddSub505/2
  Delay583/1 -> CMult606/1, Delay586/1
  Delay447/1 -> CMult472/1, Delay450/1
  Delay361/1 -> CMult378/1, Delay362/1
  Gateway In10/1 -> CMult600/1, Delay580/1
  CMult606/1 -> AddSub563/1
  Delay421/1 -> CMult440/1, Delay422/1
  AddSub526/1 -> AddSub422/2
  AddSub366/1 -> AddSub330/2
  CMult394/1 -> AddSub366/1
  Delay385/1 -> CMult409/1, Delay389/1
  CMult414/1 -> AddSub374/1
  AddSub349/1 -> AddSub387/2
  AddSub507/1 -> AddSub546/2
  AddSub255/1 -> AddSub539/2
  Delay561/1 -> CMult586/1, Delay564/1
  CMult618/1 -> AddSub416/1
  AddSub189/1 -> AddSub563/2
  CMult564/1 -> AddSub438/1
  AddSub464/1 -> AddSub529/2
  Delay607/1 -> CMult611/1, Delay591/1
  AddSub260/1 -> AddSub560/2
  AddSub241/1 -> AddSub428/2
  AddSub425/1 -> AddSub467/2
  Delay528/1 -> CMult563/1, Delay539/1
  Delay531/1 -> CMult568/1
  Delay608/1 -> CMult350/1, Delay609/1
  CMult500/1 -> AddSub447/1
  AddSub251/1 -> AddSub516/2
  From Workspace10/1 -> Gateway In10/1
  AddSub319/1 -> AddSub364/2
  CMult563/1 -> AddSub437/1
  AddSub239/1 -> AddSub416/2
  Delay513/1 -> CMult506/1, Delay514/1
  CMult357/1 -> AddSub593/1
  Gateway In13/1 -> CMult400/1, Delay380/1
  CMult573/1 -> AddSub517/1
  Delay551/1 -> CMult576/1, Delay554/1
  CMult620/1 -> AddSub439/1
  CMult365/1 -> AddSub319/1
  Delay375/1 -> CMult358/1, Delay342/1
  CMult364/1 -> AddSub318/1
  CMult602/1 -> AddSub538/1
  CMult592/1 -> AddSub502/1
  Delay594/1 -> CMult615/1, Delay595/1
  AddSub256/1 -> AddSub550/2
  AddSub248/1 -> AddSub494/2
  Delay354/1 -> CMult379/1, Delay363/1
  Delay422/1 -> CMult449/1, Delay431/1
  AddSub245/1 -> AddSub461/2
  Delay367/1 -> CMult389/1, Delay372/1
  AddSub257/1 -> AddSub557/2
  AddSub339/1 -> AddSub568/2
  Delay342/1 -> CMult359/1, Delay343/1
  Delay568/1 -> CMult591/1, Delay569/1
  AddSub369/1 -> AddSub414/2
  Gateway In17/1 -> CMult510/1, Delay484/1
  CMult388/1 -> AddSub588/1
  CMult582/1 -> AddSub440/1
  AddSub258/1 -> AddSub558/2
  CMult362/1 -> AddSub589/1
  AddSub552/1 -> AddSub447/2
  AddSub582/1 -> AddSub348/2
  CMult410/1 -> AddSub369/1
  AddSub420/1 -> AddSub460/2
  CMult356/1 -> AddSub592/1
  CMult359/1 -> AddSub321/1
  Delay360/1 -> CMult377/1, Delay361/1
  CMult444/1 -> AddSub337/1
  AddSub427/1 -> AddSub577/2
  AddSub376/1 -> AddSub488/2
  Delay502/1 -> CMult524/1, Delay498/1
  AddSub400/1 -> AddSub517/2
  AddSub247/1 -> AddSub483/2
  CMult609/1 -> AddSub317/1
  CMult431/1 -> AddSub343/1
  Delay347/1 -> CMult366/1, Delay350/1
  Delay454/1 -> CMult477/1, Delay455/1
  CMult435/1 -> AddSub364/1
  AddSub190/1 -> AddSub564/2
  Delay374/1 -> CMult357/1, Delay375/1
  AddSub592/1 -> AddSub358/2
  CMult503/1 -> AddSub451/1
  CMult389/1 -> AddSub590/1
  AddSub561/1 -> AddSub318/2
  CMult355/1 -> AddSub591/1
  AddSub538/1 -> AddSub589/2
  Delay343/1 -> CMult362/1, Delay346/1
  AddSub585/1 -> AddSub323/2
  Delay344/1 -> CMult361/1, Delay345/1
  CMult557/1 -> AddSub430/1
  Delay588/1 -> CMult604/1, Delay584/1
  Delay521/1 -> CMult549/1, Delay525/1
  Delay580/1 -> CMult601/1, Delay581/1
  Delay350/1 -> CMult367/1, Delay351/1
  AddSub394/1 -> AddSub573/2
  Gateway In11/1 -> CMult360/1, Delay344/1
  Delay441/1 -> CMult391/1, Delay442/1
  AddSub555/1 -> AddSub451/2
  Delay345/1 -> CMult372/1, Delay356/1
  AddSub372/1 -> AddSub571/2
  CMult562/1 -> AddSub436/1
  CMult366/1 -> AddSub320/1
  CMult605/1 -> AddSub562/1
  CMult363/1 -> AddSub595/1
  AddSub374/1 -> AddSub464/2
  CMult547/1 -> AddSub469/1
  CMult607/1 -> AddSub574/1
  Delay490/1 -> CMult517/1, Delay491/1
  Delay348/1 -> CMult365/1, Delay349/1
  AddSub358/1 -> AddSub397/2
  Delay372/1 -> CMult355/1, Delay373/1
  AddSub445/1 -> AddSub487/2
  Delay371/1 -> CMult371/1, Delay355/1
  AddSub457/1 -> AddSub417/2
  CMult378/1 -> AddSub576/1
  CMult629/1 -> AddSub539/1
  AddSub357/1 -> AddSub396/2
  AddSub451/1 -> AddSub493/2
  Delay409/1 -> CMult396/1, Delay410/1
  AddSub191/1 -> AddSub574/2
  Delay411/1 -> CMult398/1, Delay378/1
  Delay402/1 -> CMult424/1, Delay404/1
  Delay522/1 -> CMult547/1, Delay523/1
  AddSub450/1 -> AddSub580/2
  CMult454/1 -> AddSub349/1
  CMult450/1 -> AddSub345/1
  Delay596/1 -> CMult617/1, Delay597/1
  CMult476/1 -> AddSub406/1
  CMult586/1 -> AddSub488/1
  CMult417/1 -> AddSub378/1
  CMult595/1 -> AddSub506/1
  Delay407/1 -> CMult411/1, Delay391/1
  Delay600/1 -> CMult621/1, Delay601/1
  CMult464/1 -> AddSub521/1
  CMult426/1 -> AddSub390/1
  CMult449/1 -> AddSub344/1
  Delay412/1 -> CMult431/1, Delay413/1
  CMult382/1 -> AddSub581/1
  CMult411/1 -> AddSub370/1
  CMult458/1 -> AddSub354/1
  Delay359/1 -> CMult388/1
  Delay351/1 -> CMult368/1, Delay352/1
  CMult384/1 -> AddSub583/1
  AddSub365/1 -> AddSub329/2
  Delay535/1 -> CMult560/1, Delay536/1
  Delay591/1 -> CMult613/1, Delay593/1
  CMult372/1 -> AddSub569/1
  Delay373/1 -> CMult356/1, Delay374/1
  Delay398/1 -> CMult414/1, Delay394/1
  Delay549/1 -> CMult582/1, Delay560/1
  CMult461/1 -> AddSub513/1
  CMult361/1 -> AddSub577/1
  CMult619/1 -> AddSub428/1
  AddSub504/1 -> AddSub543/2
  CMult352/1 -> AddSub558/1
  CMult358/1 -> AddSub594/1
  CMult423/1 -> AddSub386/1
  Delay366/1 -> CMult384/1, Delay368/1
  CMult416/1 -> AddSub376/1
  Delay405/1 -> CMult426/1, Delay406/1
  CMult512/1 -> AddSub487/1
  Gateway In15/1 -> CMult470/1, Delay448/1
  AddSub252/1 -> AddSub527/2
  Delay391/1 -> CMult413/1, Delay393/1
  CMult377/1 -> AddSub575/1
  CMult409/1 -> AddSub368/1
  CMult440/1 -> AddSub333/1
  AddSub337/1 -> AddSub374/2
  CMult457/1 -> AddSub353/1
  AddSub361/1 -> AddSub570/2
  Delay537/1 -> CMult562/1, Delay538/1
  Delay356/1 -> CMult383/1, Delay367/1
  AddSub246/1 -> AddSub472/2
  CMult549/1 -> AddSub411/1
  Delay562/1 -> CMult585/1, Delay563/1
  AddSub580/1 -> AddSub346/2
  AddSub186/1 -> AddSub561/2
  AddSub443/1 -> AddSub485/2
  CMult387/1 -> AddSub587/1
  CMult398/1 -> AddSub399/1
  AddSub367/1 -> AddSub401/2
  CMult538/1 -> AddSub486/1
  CMult369/1 -> AddSub566/1
  Delay501/1 -> CMult528/1, Delay502/1
  Delay349/1 -> CMult369/1, Delay353/1
  CMult374/1 -> AddSub571/1
  Delay357/1 -> CMult376/1, Delay360/1
  CMult367/1 -> AddSub322/1
  Delay440/1 -> CMult390/1, Delay441/1
  Delay456/1 -> CMult474/1, Delay452/1
  Delay352/1 -> CMult364/1, Delay348/1
  AddSub438/1 -> AddSub480/2
  AddSub534/1 -> AddSub431/2
  Delay603/1 -> CMult629/1, Delay608/1
  CMult611/1 -> AddSub339/1
  AddSub421/1 -> AddSub462/2
  CMult373/1 -> AddSub570/1
  Delay394/1 -> CMult415/1, Delay395/1
  Delay355/1 -> CMult373/1, Delay357/1
  AddSub430/1 -> AddSub470/2
  AddSub230/1 -> AddSub339/2
  CMult413/1 -> AddSub373/1
  CMult419/1 -> AddSub381/1
  CMult407/1 -> AddSub331/1
  Delay358/1 -> CMult375/1, Delay359/1
  Delay582/1 -> CMult603/1, Delay583/1
  Delay429/1 -> CMult448/1, Delay430/1
  Delay517/1 -> CMult552/1, Delay528/1
  CMult432/1 -> AddSub355/1
  Delay393/1 -> CMult416/1, Delay396/1
  Delay362/1 -> CMult374/1, Delay358/1
  AddSub240/1 -> AddSub427/2
  Delay388/1 -> CMult404/1, Delay384/1
  Delay436/1 -> CMult455/1, Delay437/1
  AddSub424/1 -> AddSub466/2
  CMult386/1 -> AddSub586/1
  AddSub229/1 -> AddSub328/2
  Delay378/1 -> CMult399/1, Delay379/1
  CMult427/1 -> AddSub391/1
  Delay611/1 -> CMult353/1, Delay340/1
  Delay390/1 -> CMult419/1, Delay399/1
  Delay435/1 -> CMult459/1, Delay440/1
  Delay486/1 -> CMult513/1, Delay487/1
  CMult371/1 -> AddSub568/1
  AddSub560/1 -> AddSub595/2
  CMult436/1 -> AddSub365/1
  AddSub382/1 -> AddSub500/2
  Delay576/1 -> CMult460/1, Delay577/1
  CMult376/1 -> AddSub573/1
  AddSub531/1 -> AddSub429/2
  CMult459/1 -> AddSub356/1
  Gateway In12/1 -> CMult430/1, Delay412/1
  Delay415/1 -> CMult436/1, Delay418/1
  AddSub416/1 -> AddSub576/2
  Delay368/1 -> CMult385/1, Delay369/1
  CMult623/1 -> AddSub472/1
  Delay470/1 -> CMult494/1, Delay472/1
  AddSub403/1 -> AddSub454/2
  Delay397/1 -> CMult418/1, Delay398/1
  Delay369/1 -> CMult386/1, Delay370/1
  CMult622/1 -> AddSub461/1
  AddSub566/1 -> AddSub325/2
  CMult401/1 -> AddSub380/1
  Delay381/1 -> CMult412/1, Delay392/1
  Delay379/1 -> CMult402/1, Delay382/1
  AddSub238/1 -> AddSub405/2
  Delay392/1 -> CMult423/1, Delay403/1
  AddSub502/1 -> AddSub541/2
  Delay597/1 -> CMult618/1, Delay598/1
  CMult448/1 -> AddSub342/1
  Delay547/1 -> CMult503/1, Delay480/1
  From Workspace11/1 -> Gateway In11/1
  From Workspace13/1 -> Gateway In13/1
  CMult626/1 -> AddSub505/1
  Delay526/1 -> CMult559/1, Delay535/1
  AddSub345/1 -> AddSub382/2
  CMult637/1 -> AddSub624/1
  AddSub493/1 -> AddSub629/2
  ? -> Delay628/1
  ? -> CMult649/1
  AddSub460/1 -> AddSub604/2
  AddSub467/1 -> AddSub609/2
  CMult651/1 -> AddSub610/1
  CMult664/1 -> AddSub625/1
  Delay634/1 -> CMult656/1, Delay635/1
  AddSub487/1 -> AddSub624/2
  Delay633/1 -> CMult655/1, Delay634/1
  CMult658/1 -> AddSub618/1
  AddSub468/1 -> AddSub610/2
  ? -> CMult657/1
  CMult646/1 -> AddSub605/1
  AddSub491/1 -> AddSub627/2
  CMult657/1 -> AddSub617/1
  AddSub413/1 -> AddSub597/2
  CMult653/1 -> AddSub612/1
  CMult659/1 -> AddSub619/1
  ? -> CMult641/1
  ? -> Delay620/1
  Delay629/1 -> CMult663/1
  ? -> Delay639/1
  ? -> CMult660/1
  AddSub474/1 -> AddSub614/2
  AddSub495/1 -> AddSub630/2
  Gateway In18/1 -> Delay614/1, CMult635/1
  AddSub478/1 -> AddSub617/2
  AddSub477/1 -> AddSub616/2
  ? -> CMult642/1
  AddSub484/1 -> AddSub621/2
  AddSub471/1 -> AddSub612/2
  CMult632/1 -> AddSub628/1
  AddSub481/1 -> AddSub620/2
  AddSub486/1 -> AddSub623/2
  Delay640/1 -> CMult662/1, Delay641/1
  AddSub412/1 -> AddSub596/2
  CMult641/1 -> AddSub598/1
  CMult649/1 -> AddSub608/1
  ? -> Delay621/1
  CMult636/1 -> AddSub613/1
  CMult652/1 -> AddSub611/1
  CMult647/1 -> AddSub606/1
  CMult634/1 -> AddSub599/1
  Delay630/1 -> CMult652/1, Delay631/1
  Delay637/1 -> CMult664/1, Delay642/1
  ? -> Delay622/1
  ? -> CMult643/1
  Delay614/1 -> CMult636/1, Delay615/1
  AddSub459/1 -> AddSub603/2
  AddSub463/1 -> AddSub606/2
  CMult655/1 -> AddSub615/1
  Delay644/1 -> CMult632/1, Delay645/1
  Delay618/1 -> CMult640/1, Delay619/1
  CMult639/1 -> AddSub596/1
  AddSub473/1 -> AddSub613/2
  ? -> CMult630/1
  CMult640/1 -> AddSub597/1
  Delay639/1 -> CMult661/1, Delay640/1
  AddSub458/1 -> AddSub602/2
  AddSub418/1 -> AddSub600/2
  CMult631/1 -> AddSub627/1
  ? -> Delay643/1
  AddSub479/1 -> AddSub618/2
  CMult638/1 -> AddSub630/1
  Delay616/1 -> CMult638/1, Delay617/1
  AddSub466/1 -> AddSub608/2
  AddSub462/1 -> AddSub605/2
  AddSub480/1 -> AddSub619/2
  ? -> Delay632/1
  AddSub485/1 -> AddSub622/2
  CMult663/1 -> AddSub623/1
  CMult630/1 -> AddSub626/1
  AddSub470/1 -> AddSub611/2
  Delay615/1 -> CMult647/1, Delay626/1
  CMult635/1 -> AddSub602/1
  CMult660/1 -> AddSub620/1
  ? -> CMult633/1
  ? -> Delay630/1
  AddSub419/1 -> AddSub601/2
  ? -> CMult651/1
  Delay643/1 -> CMult631/1, Delay644/1
  ? -> CMult644/1
  CMult645/1 -> AddSub604/1
  CMult656/1 -> AddSub616/1
  ? -> Delay612/1
  CMult650/1 -> AddSub609/1
  ? -> CMult659/1
  ? -> Delay638/1
  AddSub465/1 -> AddSub607/2
  Delay622/1 -> CMult639/1, Delay618/1
  CMult643/1 -> AddSub601/1
  ? -> CMult646/1
  ? -> Delay625/1
  AddSub415/1 -> AddSub598/2
  AddSub417/1 -> AddSub599/2
  ? -> Delay627/1
  ? -> CMult648/1
  AddSub490/1 -> AddSub626/2
  CMult642/1 -> AddSub600/1
  ? -> Delay629/1
  ? -> CMult650/1
  CMult654/1 -> AddSub614/1
  CMult662/1 -> AddSub622/1
  ? -> Delay623/1
  ? -> CMult634/1
  ? -> Delay613/1
  CMult633/1 -> AddSub629/1
  CMult648/1 -> AddSub607/1
  ? -> Delay633/1
  ? -> Delay616/1
  CMult661/1 -> AddSub621/1
  ? -> CMult653/1
  AddSub489/1 -> AddSub625/2
  From Workspace18/1 -> Gateway In18/1
  ? -> CMult637/1
  AddSub475/1 -> AddSub615/2
  ? -> Delay624/1
  Delay626/1 -> CMult658/1, Delay637/1
  ? -> Delay636/1
  ? -> CMult645/1
  CMult644/1 -> AddSub603/1
  ? -> CMult654/1
  AddSub492/1 -> AddSub628/2
